simulink model "PresentationNetworkOrgignalparametrs3Copter"  (R2020a)
settings: Solver=FixedStepAuto  StartTime=0.0  StopTime=0.1  FixedStep=0.01  RelTol=1e-3
values from neighbouring files (symbols this model uses):
  Te = 0.012    [4двигателядообученный.mat]    (also in deepLearning.m; tdeepLearning.m)
  Tm = 0.025    [4двигателядообученный.mat]    (also in deepLearning.m; tdeepLearning.m)
  x1 = 1    [4двигателядообученный.mat]
  x2 = 1    [4двигателядообученный.mat]
  x3 = 1    [4двигателядообученный.mat]
undefined symbols (not defined in the file or in its folder): a1, a2, a3, a4, a5, b, d
libraries: simulink x3, dspsrcs4 x2, rllib x1
settings Model: Creator=xreno  LastModifiedBy=xreno

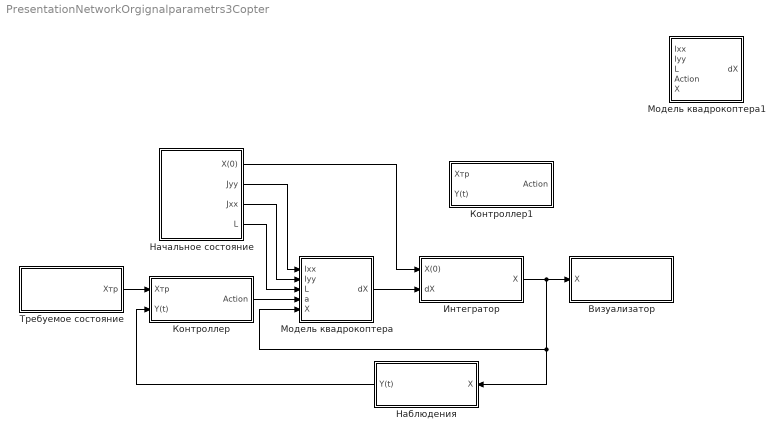
== system PresentationNetworkOrgignalparametrs3Copter ==
  Визуализатор : Subsystem
  Интегратор : Subsystem
  Контроллер : Subsystem
  Контроллер1 : Subsystem
  Модель квадрокоптера : Subsystem
  Модель квадрокоптера1 : Subsystem
  Наблюдения : Subsystem
  Начальное состояние : Subsystem
  Требуемое состояние : Subsystem
  wires:
  Начальное состояние/2(Jyy) -> Модель квадрокоптера/1(Ixx)
  Начальное состояние/1(X(0)) -> Интегратор/1(X(0))
  Модель квадрокоптера/1(dX) -> Интегратор/2(dX)
  Требуемое состояние/1(Xтр) -> Контроллер/1(Xтр)
  Интегратор/1(X) -> Наблюдения/1(X), Модель квадрокоптера/5(X), Визуализатор/1(X)
  Начальное состояние/3(Jxx) -> Модель квадрокоптера/2(Iyy)
  Наблюдения/1(Y(t)) -> Контроллер/2(Y(t))
  Начальное состояние/4(L) -> Модель квадрокоптера/3(L)
  Контроллер/1(Action) -> Модель квадрокоптера/4(a)

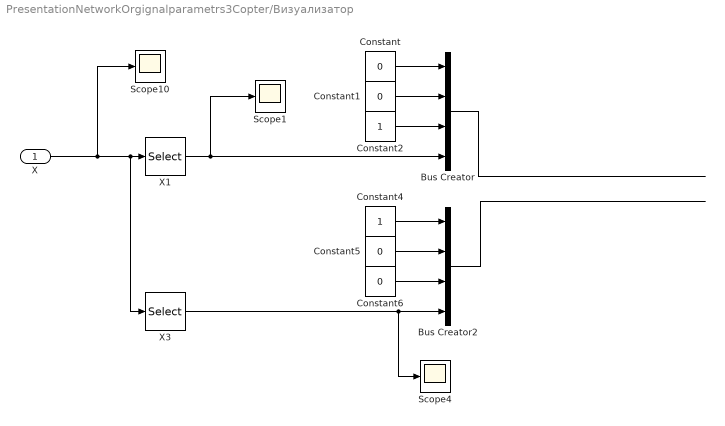
== system PresentationNetworkOrgignalparametrs3Copter/Визуализатор ==
  X : Inport
  Bus Creator : BusCreator  Inputs=4
  Bus Creator2 : BusCreator  Inputs=4
  Constant{,1,5..6} (4 alike) : Constant  Value=0
  Constant2 : Constant
  Constant4 : Constant
  Scope1 : Scope
  Scope10 : Scope
  Scope4 : Scope
  X1 : Selector  InputPortWidth=6  IndexOptions=Index vector (dialog)  Indices=[1]  OutputSizes=1
  X3 : Selector  InputPortWidth=6  IndexOptions=Index vector (dialog)  Indices=[3]  OutputSizes=1
  wires:
  Constant5/1 -> Bus Creator2/2
  Constant4/1 -> Bus Creator2/1
  Constant1/1 -> Bus Creator/2
  Bus Creator2/1 -> ?
  Constant6/1 -> Bus Creator2/3
  Constant2/1 -> Bus Creator/3
  Constant/1 -> Bus Creator/1
  Bus Creator/1 -> ?
  X/1 -> Scope10/1, X3/1, X1/1
  X1/1 -> Bus Creator/4, Scope1/1
  X3/1 -> Scope4/1, Bus Creator2/4

== system PresentationNetworkOrgignalparametrs3Copter/Интегратор ==
  X(0) : Inport
  dX : Inport  Port=2
  Integrator2 : Integrator  InitialConditionSource=external
  X : Outport
  wires:
  X(0)/1 -> Integrator2/2
  dX/1 -> Integrator2/1
  Integrator2/1 -> X/1

== system PresentationNetworkOrgignalparametrs3Copter/Контроллер ==
  Xтр : Inport
  Y(t) : Inport  Port=2
  Product2 : Product
  Rate Transition1 : RateTransition
  Rate Transition2 : RateTransition
  Rate Transition5 : RateTransition
  s1 : Constant  Value=8
  Блок RL Agent : rllib/RL Agent  Agent=agent  ProvideReward=on  ProvideIsDone=on  ProvideCumRwd=off  TreatAsDirectFeedthrough=on  CollectLoggedSignals=on  CollectModelStates=on
  Калькулятор награды : Subsystem
  Регулируемые параметры : Subsystem
  Action : Outport
  wires:
  Калькулятор награды/1(Reward) -> Rate Transition1/1
  Калькулятор награды/2(IsDone) -> Rate Transition2/1
  Product2/1 -> Action/1
  Регулируемые параметры/1(Z) -> Rate Transition5/1, Калькулятор награды/1(X)
  Блок RL Agent/1 -> Product2/2
  s1/1 -> Product2/1
  Rate Transition5/1 -> Блок RL Agent/1
  Rate Transition1/1 -> Блок RL Agent/2
  Rate Transition2/1 -> Блок RL Agent/3
  Y(t)/1 -> Регулируемые параметры/1(Y)
  Xтр/1 -> Регулируемые параметры/2(XT)

== system PresentationNetworkOrgignalparametrs3Copter/Контроллер1 ==
  Xтр : Inport
  Y(t) : Inport  Port=2
  Mux : Mux  Inputs=3
  PID-регулятор по крену : simulink/Continuous/PID Controller  Controller=PID  Form=Parallel  TimeDomain=Continuous-time  UseExternalTs=off  SampleTime=-1  IntegratorMethod=Forward Euler  FilterMethod=Forward Euler  ControllerParametersSource=internal  P=1  I=1  D=0  UseFilter=on  N=100  TunerSelectOption=Transfer Function Based (PID Tuner App)  InitialConditionSource=internal  InitialConditionForIntegrator=0  InitialConditionForFilter=0  DifferentiatorICPrevScaledInput=0  ExternalReset=none  TrackingMode=off  Kt=1  LimitOutput=off  UpperSaturationLimit=inf  LowerSaturationLimit=-inf  LinearizeAsGain=on  AntiWindupMode=none  Kb=1  POutMin=[]  POutMax=[]  IOutMin=[]  IOutMax=[]  DOutMin=[]  DOutMax=[]  NOutMin=[]  NOutMax=[]  SumOutMin=[]  SumOutMax=[]  SaturationOutMin=[]  SaturationOutMax=[]  PParamMin=[]  PParamMax=[]  IParamMin=[]  IParamMax=[]  DParamMin=[]  DParamMax=[]  NParamMin=[]  NParamMax=[]  KbParamMin=[]  KbParamMax=[]  KtParamMin=[]  KtParamMax=[]  KbOutMin=[]  KbOutMax=[]  KtOutMin=[]  KtOutMax=[]  IntegratorOutMin=[]  IntegratorOutMax=[]  FilterOutMin=[]  FilterOutMax=[]  SumI1OutMin=[]  SumI1OutMax=[]  SumI2OutMin=[]  SumI2OutMax=[]  SumI3OutMin=[]  SumI3OutMax=[]  SumI4OutMin=[]  SumI4OutMax=[]  SumDOutMin=[]  SumDOutMax=[]  DifferentiatorOutMin=[]  DifferentiatorOutMax=[]  FilterDiffOutCoefMin=[]  FilterDiffOutCoefMax=[]  ReciprocalOutMin=[]  ReciprocalOutMax=[]  SumDenOutMin=[]  SumDenOutMax=[]  SumNumOutMin=[]  SumNumOutMax=[]  DivideOutMin=[]  DivideOutMax=[]  UdiffTsProdOutMin=[]  UdiffTsProdOutMax=[]  NTsProdOutMin=[]  NTsProdOutMax=[]  UintegralTsProdOutMin=[]  UintegralTsProdOutMax=[]  UngainTsProdOutMin=[]  UngainTsProdOutMax=[]  IntegratorContinuousStateAttributes=''  IntegratorStateMustResolveToSignalObject=off  IntegratorRTWStateStorageClass=Auto  FilterContinuousStateAttributes=''  FilterStateMustResolveToSignalObject=off  FilterRTWStateStorageClass=Auto  ParallelPVariant=InternalParameters  IdealPVariant=Disabled  IVariant=InternalParameters  DVariant=InternalParameters  IntegratorVariant=Continuous  SatVariant=Disabled  AWVariant=Passthrough  PCopyVariant=Disabled  TRVariant=Disabled  FdbkBlocksVariant=Forward  IdealPFdbkVariant=Disabled  SatFdbkVariant=Disabled  DerivativeFilterVariant=ContFilter  NVariant=InternalParameters  NCopyVariant=Disabled  FilterICVariant=InternalICsFilter  IntegratorICVariant=InternalICs  ExternalResetVariant=Disabled  TRSumVariant=Passthrough  SumFdbkVariant=Disabled  SumVariant=Sum_PID  TsampFilterVariant=InternalTs  TsampNgainVariant=Passthrough  TsampIntegralVariant=Passthrough
  PID-регулятор по рысканью : simulink/Continuous/PID Controller  Controller=PID  Form=Parallel  TimeDomain=Continuous-time  UseExternalTs=off  SampleTime=-1  IntegratorMethod=Forward Euler  FilterMethod=Forward Euler  ControllerParametersSource=internal  P=1  I=1  D=0  UseFilter=on  N=100  TunerSelectOption=Transfer Function Based (PID Tuner App)  InitialConditionSource=internal  InitialConditionForIntegrator=0  InitialConditionForFilter=0  DifferentiatorICPrevScaledInput=0  ExternalReset=none  TrackingMode=off  Kt=1  LimitOutput=off  UpperSaturationLimit=inf  LowerSaturationLimit=-inf  LinearizeAsGain=on  AntiWindupMode=none  Kb=1  POutMin=[]  POutMax=[]  IOutMin=[]  IOutMax=[]  DOutMin=[]  DOutMax=[]  NOutMin=[]  NOutMax=[]  SumOutMin=[]  SumOutMax=[]  SaturationOutMin=[]  SaturationOutMax=[]  PParamMin=[]  PParamMax=[]  IParamMin=[]  IParamMax=[]  DParamMin=[]  DParamMax=[]  NParamMin=[]  NParamMax=[]  KbParamMin=[]  KbParamMax=[]  KtParamMin=[]  KtParamMax=[]  KbOutMin=[]  KbOutMax=[]  KtOutMin=[]  KtOutMax=[]  IntegratorOutMin=[]  IntegratorOutMax=[]  FilterOutMin=[]  FilterOutMax=[]  SumI1OutMin=[]  SumI1OutMax=[]  SumI2OutMin=[]  SumI2OutMax=[]  SumI3OutMin=[]  SumI3OutMax=[]  SumI4OutMin=[]  SumI4OutMax=[]  SumDOutMin=[]  SumDOutMax=[]  DifferentiatorOutMin=[]  DifferentiatorOutMax=[]  FilterDiffOutCoefMin=[]  FilterDiffOutCoefMax=[]  ReciprocalOutMin=[]  ReciprocalOutMax=[]  SumDenOutMin=[]  SumDenOutMax=[]  SumNumOutMin=[]  SumNumOutMax=[]  DivideOutMin=[]  DivideOutMax=[]  UdiffTsProdOutMin=[]  UdiffTsProdOutMax=[]  NTsProdOutMin=[]  NTsProdOutMax=[]  UintegralTsProdOutMin=[]  UintegralTsProdOutMax=[]  UngainTsProdOutMin=[]  UngainTsProdOutMax=[]  IntegratorContinuousStateAttributes=''  IntegratorStateMustResolveToSignalObject=off  IntegratorRTWStateStorageClass=Auto  FilterContinuousStateAttributes=''  FilterStateMustResolveToSignalObject=off  FilterRTWStateStorageClass=Auto  ParallelPVariant=InternalParameters  IdealPVariant=Disabled  IVariant=InternalParameters  DVariant=InternalParameters  IntegratorVariant=Continuous  SatVariant=Disabled  AWVariant=Passthrough  PCopyVariant=Disabled  TRVariant=Disabled  FdbkBlocksVariant=Forward  IdealPFdbkVariant=Disabled  SatFdbkVariant=Disabled  DerivativeFilterVariant=ContFilter  NVariant=InternalParameters  NCopyVariant=Disabled  FilterICVariant=InternalICsFilter  IntegratorICVariant=InternalICs  ExternalResetVariant=Disabled  TRSumVariant=Passthrough  SumFdbkVariant=Disabled  SumVariant=Sum_PID  TsampFilterVariant=InternalTs  TsampNgainVariant=Passthrough  TsampIntegralVariant=Passthrough
  PID-регулятор по тангажу : simulink/Continuous/PID Controller  Controller=PID  Form=Parallel  TimeDomain=Continuous-time  UseExternalTs=off  SampleTime=-1  IntegratorMethod=Forward Euler  FilterMethod=Forward Euler  ControllerParametersSource=internal  P=1  I=1  D=0  UseFilter=on  N=100  TunerSelectOption=Transfer Function Based (PID Tuner App)  InitialConditionSource=internal  InitialConditionForIntegrator=0  InitialConditionForFilter=0  DifferentiatorICPrevScaledInput=0  ExternalReset=none  TrackingMode=off  Kt=1  LimitOutput=off  UpperSaturationLimit=inf  LowerSaturationLimit=-inf  LinearizeAsGain=on  AntiWindupMode=none  Kb=1  POutMin=[]  POutMax=[]  IOutMin=[]  IOutMax=[]  DOutMin=[]  DOutMax=[]  NOutMin=[]  NOutMax=[]  SumOutMin=[]  SumOutMax=[]  SaturationOutMin=[]  SaturationOutMax=[]  PParamMin=[]  PParamMax=[]  IParamMin=[]  IParamMax=[]  DParamMin=[]  DParamMax=[]  NParamMin=[]  NParamMax=[]  KbParamMin=[]  KbParamMax=[]  KtParamMin=[]  KtParamMax=[]  KbOutMin=[]  KbOutMax=[]  KtOutMin=[]  KtOutMax=[]  IntegratorOutMin=[]  IntegratorOutMax=[]  FilterOutMin=[]  FilterOutMax=[]  SumI1OutMin=[]  SumI1OutMax=[]  SumI2OutMin=[]  SumI2OutMax=[]  SumI3OutMin=[]  SumI3OutMax=[]  SumI4OutMin=[]  SumI4OutMax=[]  SumDOutMin=[]  SumDOutMax=[]  DifferentiatorOutMin=[]  DifferentiatorOutMax=[]  FilterDiffOutCoefMin=[]  FilterDiffOutCoefMax=[]  ReciprocalOutMin=[]  ReciprocalOutMax=[]  SumDenOutMin=[]  SumDenOutMax=[]  SumNumOutMin=[]  SumNumOutMax=[]  DivideOutMin=[]  DivideOutMax=[]  UdiffTsProdOutMin=[]  UdiffTsProdOutMax=[]  NTsProdOutMin=[]  NTsProdOutMax=[]  UintegralTsProdOutMin=[]  UintegralTsProdOutMax=[]  UngainTsProdOutMin=[]  UngainTsProdOutMax=[]  IntegratorContinuousStateAttributes=''  IntegratorStateMustResolveToSignalObject=off  IntegratorRTWStateStorageClass=Auto  FilterContinuousStateAttributes=''  FilterStateMustResolveToSignalObject=off  FilterRTWStateStorageClass=Auto  ParallelPVariant=InternalParameters  IdealPVariant=Disabled  IVariant=InternalParameters  DVariant=InternalParameters  IntegratorVariant=Continuous  SatVariant=Disabled  AWVariant=Passthrough  PCopyVariant=Disabled  TRVariant=Disabled  FdbkBlocksVariant=Forward  IdealPFdbkVariant=Disabled  SatFdbkVariant=Disabled  DerivativeFilterVariant=ContFilter  NVariant=InternalParameters  NCopyVariant=Disabled  FilterICVariant=InternalICsFilter  IntegratorICVariant=InternalICs  ExternalResetVariant=Disabled  TRSumVariant=Passthrough  SumFdbkVariant=Disabled  SumVariant=Sum_PID  TsampFilterVariant=InternalTs  TsampNgainVariant=Passthrough  TsampIntegralVariant=Passthrough
  Scope : Scope
  Scope1 : Scope
  Selector1 : Selector  InputPortWidth=6  IndexOptions=Index vector (dialog)  Indices=[1]  OutputSizes=1
  Selector2 : Selector  InputPortWidth=6  IndexOptions=Index vector (dialog)  Indices=[3]  OutputSizes=1
  Selector3 : Selector  InputPortWidth=6  IndexOptions=Index vector (dialog)  Indices=[5]  OutputSizes=1
  Калькулятор награды : Subsystem
  Регулируемые параметры : Subsystem
  Action : Outport
  wires:
  Калькулятор награды/1(Reward) -> Scope/1
  Калькулятор награды/2(IsDone) -> Scope1/1
  Mux/1 -> Action/1
  Регулируемые параметры/1(Z) -> Калькулятор награды/1(X), Selector3/1, Selector1/1, Selector2/1
  Y(t)/1 -> Регулируемые параметры/1(Y)
  Xтр/1 -> Регулируемые параметры/2(XT)
  Selector1/1 -> PID-регулятор по крену/1
  Selector2/1 -> PID-регулятор по тангажу/1
  Selector3/1 -> PID-регулятор по рысканью/1
  PID-регулятор по тангажу/1 -> Mux/2
  PID-регулятор по крену/1 -> Mux/1
  PID-регулятор по рысканью/1 -> Mux/3

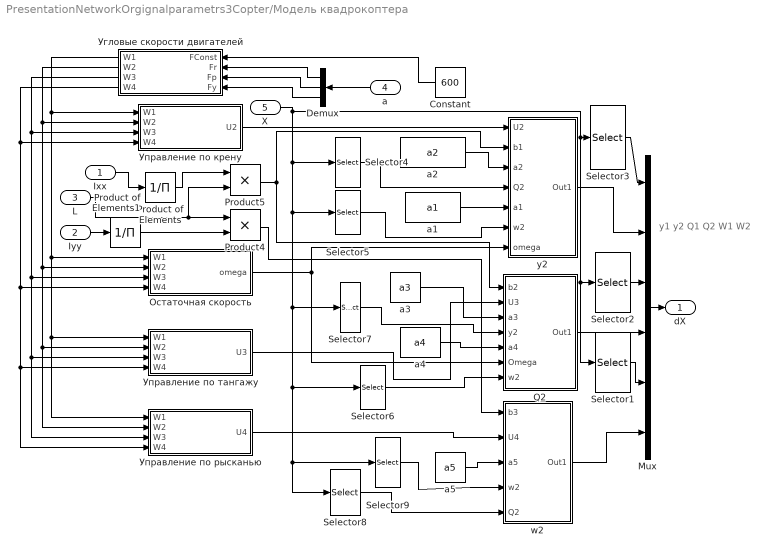
== system PresentationNetworkOrgignalparametrs3Copter/Модель квадрокоптера ==
  note: y1
      | y2
      | Q1
      | Q2
      | W1
      | W2
  Ixx : Inport
  Iyy : Inport  Port=2
  L : Inport  Port=3
  a : Inport  Port=4
  X : Inport  Port=5
  Constant : Constant  Value=600
  Demux : Demux  Outputs=3
  Mux : Mux  Inputs=6
  Product of Elements : Product  Inputs=/
  Product of Elements1 : Product  Inputs=/
  Product4 : Product
  Product5 : Product
  Q2 : Subsystem
  Selector{1,5..6,9} (4 alike) : Selector  InputPortWidth=6  IndexOptions=Index vector (dialog)  Indices=[6]  OutputSizes=1
  Selector2 : Selector  InputPortWidth=6  IndexOptions=Index vector (dialog)  Indices=[4]  OutputSizes=1
  Selector3 : Selector  InputPortWidth=6  IndexOptions=Index vector (dialog)  Indices=[2]  OutputSizes=1
  Selector4 : Selector  InputPortWidth=6  IndexOptions=Index vector (dialog)  Indices=[4]  OutputSizes=1
  Selector7 : Selector  InputPortWidth=6  IndexOptions=Index vector (dialog)  Indices=[2]  OutputSizes=1
  Selector8 : Selector  InputPortWidth=6  IndexOptions=Index vector (dialog)  Indices=[4]  OutputSizes=1
  a1 : Constant  Value=a1
  a2 : Constant  Value=a2
  a3 : Constant  Value=a3
  a4 : Constant  Value=a4
  a5 : Constant  Value=a5
  w2 : Subsystem
  y2 : Subsystem
  Остаточная скорость : Subsystem
  Угловые скорости двигателей : Subsystem
  Управление по крену : Subsystem
  Управление по рысканью : Subsystem
  Управление по тангажу : Subsystem
  dX : Outport
  wires:
  X/1 -> Selector3/1, Selector1/1, Selector2/1, Selector6/1, Selector9/1, Selector8/1, Selector7/1, Selector5/1, Selector4/1
  a/1 -> Demux/1
  Mux/1 -> dX/1
  Constant/1 -> Угловые скорости двигателей/1(FConst)
  Угловые скорости двигателей/2(W2) -> Управление по рысканью/2(W2), Управление по тангажу/2(W2), Остаточная скорость/2(W2), Управление по крену/2(W2)
  Угловые скорости двигателей/4(W4) -> Управление по рысканью/4(W4), Управление по тангажу/4(W4), Остаточная скорость/4(W4), Управление по крену/4(W4)
  Угловые скорости двигателей/3(W3) -> Управление по рысканью/3(W3), Управление по тангажу/3(W3), Остаточная скорость/3(W3), Управление по крену/3(W3)
  Управление по крену/1(U2) -> y2/1(U2)
  Product5/1 -> y2/2(b1), Q2/1(b2)
  Управление по тангажу/1(U3) -> Q2/2(U3)
  Product of Elements/1 -> Product5/1
  Product of Elements1/1 -> Product4/2
  Product4/1 -> w2/1(b3)
  L/1 -> Product5/2, Product4/1
  Iyy/1 -> Product of Elements1/1
  Ixx/1 -> Product of Elements/1
  Угловые скорости двигателей/1(W1) -> Управление по рысканью/1(W1), Управление по тангажу/1(W1), Остаточная скорость/1(W1), Управление по крену/1(W1)
  Demux/1 -> Угловые скорости двигателей/2(Fr)
  Demux/2 -> Угловые скорости двигателей/3(Fp)
  y2/1(Out1) -> Mux/2
  Q2/1(Out1) -> Mux/4
  w2/1(Out1) -> Mux/6
  Selector3/1 -> Mux/1
  Selector2/1 -> Mux/3
  Selector1/1 -> Mux/5
  Остаточная скорость/1(omega) -> y2/7(omega), Q2/6(Omega)
  a3/1 -> Q2/3(a3)
  a1/1 -> y2/5(a1)
  a2/1 -> y2/3(a2)
  a4/1 -> Q2/5(a4)
  a5/1 -> w2/3(a5)
  Управление по рысканью/1(U4) -> w2/2(U4)
  Selector4/1 -> y2/4(Q2)
  Selector5/1 -> y2/6(w2)
  Selector6/1 -> Q2/7(w2)
  Selector7/1 -> Q2/4(y2)
  Selector8/1 -> w2/5(Q2)
  Selector9/1 -> w2/4(w2)
  Demux/3 -> Угловые скорости двигателей/4(Fy)

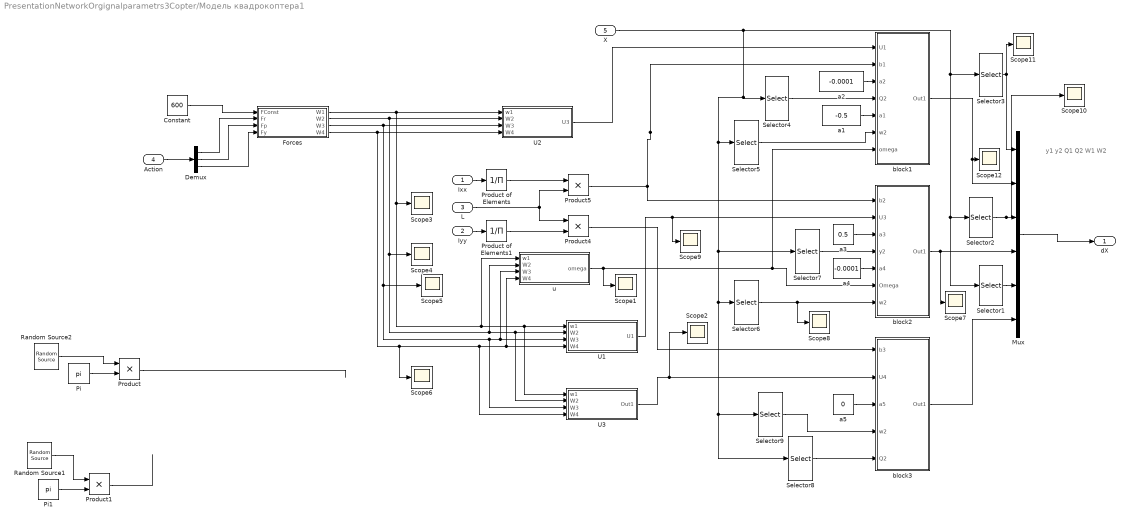
== system PresentationNetworkOrgignalparametrs3Copter/Модель квадрокоптера1 ==
  note: y1
      | y2
      | Q1
      | Q2
      | W1
      | W2
  Ixx : Inport
  Iyy : Inport  Port=2
  L : Inport  Port=3
  Action : Inport  Port=4
  X : Inport  Port=5
  Constant : Constant  Value=600
  Demux : Demux  Outputs=3
  Forces : Subsystem
  Mux : Mux  Inputs=6
  Pi : Constant  Value=pi  OutDataTypeStr=Inherit: Inherit via back propagation
  Pi1 : Constant  Value=pi  OutDataTypeStr=Inherit: Inherit via back propagation
  Product{,1,4..5} (4 alike) : Product
  Product of Elements : Product  Inputs=/
  Product of Elements1 : Product  Inputs=/
  Random Source1 : dspsrcs4/Random Source  SrcType=Uniform  NormMethod=Ziggurat  CltLength=12  MinVal=-1  MaxVal=1  MeanVal=0  VarVal=1  RepMode=Not repeatable  rawSeed=1  IsInherit=off  SampMode=Discrete  SampTime=1  SampFrame=1  DataType=Double  OutComplex=Real  OutputFrames=off
  Random Source2 : dspsrcs4/Random Source  SrcType=Uniform  NormMethod=Ziggurat  CltLength=12  MinVal=-1  MaxVal=1  MeanVal=0  VarVal=1  RepMode=Not repeatable  rawSeed=1  IsInherit=off  SampMode=Discrete  SampTime=1  SampFrame=1  DataType=Double  OutComplex=Real  OutputFrames=off
  Scope{1..12} (12 alike) : Scope
  Selector{1,5..6,9} (4 alike) : Selector  InputPortWidth=6  IndexOptions=Index vector (dialog)  Indices=[6]  OutputSizes=1
  Selector2 : Selector  InputPortWidth=6  IndexOptions=Index vector (dialog)  Indices=[4]  OutputSizes=1
  Selector3 : Selector  InputPortWidth=6  IndexOptions=Index vector (dialog)  Indices=[2]  OutputSizes=1
  Selector4 : Selector  InputPortWidth=6  IndexOptions=Index vector (dialog)  Indices=[4]  OutputSizes=1
  Selector7 : Selector  InputPortWidth=6  IndexOptions=Index vector (dialog)  Indices=[2]  OutputSizes=1
  Selector8 : Selector  InputPortWidth=6  IndexOptions=Index vector (dialog)  Indices=[4]  OutputSizes=1
  U1 : Subsystem
  U2 : Subsystem
  U3 : Subsystem
  a1 : Constant  Value=-0.5
  a2 : Constant  Value=-0.0001
  a3 : Constant  Value=0.5
  a4 : Constant  Value=-0.0001
  a5 : Constant  Value=0
  block1 : Subsystem
  block2 : Subsystem
  block3 : Subsystem
  u : Subsystem
  dX : Outport
  wires:
  X/1 -> Selector7/1, Selector8/1, Selector9/1, Selector6/1, Selector5/1, Selector4/1, Selector1/1, Selector2/1, Selector3/1
  Action/1 -> Demux/1
  Mux/1 -> dX/1
  Constant/1 -> Forces/1(FConst)
  Forces/2(W2) -> U2/2(W2), Scope4/1, u/2(W2), U1/2(W2), U3/2(W2)
  Forces/4(W4) -> U2/4(W4), Scope6/1, U3/4(W4), u/4(W4), U1/4(W4)
  Forces/3(W3) -> U2/3(W3), U3/3(W3), u/3(W3), U1/3(W3), Scope5/1
  U2/1(U3) -> block1/1(U1)
  Product5/1 -> block1/2(b1), block2/1(b2)
  U1/1(U1) -> Scope9/1, block2/2(U3)
  Product of Elements/1 -> Product5/1
  Product of Elements1/1 -> Product4/2
  Product4/1 -> block3/1(b3)
  L/1 -> Product4/1, Product5/2
  Iyy/1 -> Product of Elements1/1
  Ixx/1 -> Product of Elements/1
  Forces/1(W1) -> U2/1(w1), u/1(w1), U1/1(w1), U3/1(w1), Scope3/1
  Demux/1 -> Forces/2(Fr)
  Demux/2 -> Forces/3(Fp)
  block1/1(Out1) -> Scope12/1, Mux/2
  block2/1(Out1) -> Scope7/1, Mux/4
  block3/1(Out1) -> Mux/6
  Selector3/1 -> Scope11/1, Mux/1
  Selector2/1 -> Scope10/1, Mux/3
  Selector1/1 -> Mux/5
  u/1(omega) -> Scope1/1, block2/6(Omega), block1/7(omega)
  a3/1 -> block2/3(a3)
  a1/1 -> block1/5(a1)
  a2/1 -> block1/3(a2)
  a4/1 -> block2/5(a4)
  a5/1 -> block3/3(a5)
  U3/1(Out1) -> Scope2/1, block3/2(U4)
  Selector4/1 -> block1/4(Q2)
  Selector5/1 -> block1/6(w2)
  Selector6/1 -> Scope8/1, block2/7(w2)
  Selector7/1 -> block2/4(y2)
  Selector8/1 -> block3/5(Q2)
  Selector9/1 -> block3/4(w2)
  Demux/3 -> Forces/4(Fy)
  Pi1/1 -> Product1/2
  Product1/1 -> ?
  Pi/1 -> Product/2
  Random Source2/1 -> Product/1
  Random Source1/1 -> Product1/1
  Product/1 -> ?

== system PresentationNetworkOrgignalparametrs3Copter/Наблюдения ==
  X : Inport
  Demux : Demux  Outputs=6
  FucncN2 : MATLAB Function  TreatAsAtomicUnit=on
  FuncN1 : MATLAB Function  TreatAsAtomicUnit=on
  FuncN3 : MATLAB Function  TreatAsAtomicUnit=on
  Mux : Mux  Inputs=6
  Rate Transition{1,3..4,7} (4 alike) : RateTransition
  Y(t) : Outport
  wires:
  Mux/1 -> Y(t)/1
  Demux/3 -> FucncN2/1(inputArg1)
  FucncN2/1(outputArg1) -> Rate Transition1/1
  Rate Transition3/1 -> Mux/1
  Demux/2 -> Mux/2
  Demux/4 -> Mux/4
  X/1 -> Rate Transition4/1
  Rate Transition7/1 -> Mux/5
  Demux/5 -> FuncN3/1(inputArg1)
  Demux/6 -> Mux/6
  FuncN1/1(outputArg1) -> Rate Transition3/1
  Demux/1 -> FuncN1/1(inputArg1)
  Rate Transition4/1 -> Demux/1
  ? -> ?
  FuncN3/1(outputArg1) -> Rate Transition7/1
  Rate Transition1/1 -> Mux/3

== system PresentationNetworkOrgignalparametrs3Copter/Начальное состояние ==
  Constant1 : Constant  Value=0
  Constant2 : Constant  Value=x2
  Constant3 : Constant  Value=0
  Constant4 : Constant  Value=x1
  Constant5 : Constant  Value=x3
  Constant6 : Constant  Value=0
  Ixx : Constant
  Iyy : Constant
  L1 : Constant  Value=0.5
  Mux1 : Mux  Inputs=6
  X(0) : Outport
  Jyy : Outport  Port=2
  Jxx : Outport  Port=3
  L : Outport  Port=4
  wires:
  Constant1/1 -> Mux1/2
  Mux1/1 -> X(0)/1
  Constant3/1 -> Mux1/4
  Ixx/1 -> Jxx/1
  Iyy/1 -> Jyy/1
  L1/1 -> L/1
  Constant2/1 -> Mux1/3
  Constant4/1 -> Mux1/1
  Constant5/1 -> Mux1/5
  Constant6/1 -> Mux1/6

== system PresentationNetworkOrgignalparametrs3Copter/Требуемое состояние ==
  Constant{,1..5} (6 alike) : Constant  Value=0
  Mux1 : Mux  Inputs=6
  Xтр : Outport
  wires:
  Constant/1 -> Mux1/1
  Constant3/1 -> Mux1/4
  Constant1/1 -> Mux1/2
  Mux1/1 -> Xтр/1
  Constant2/1 -> Mux1/3
  Constant5/1 -> Mux1/6
  Constant4/1 -> Mux1/5

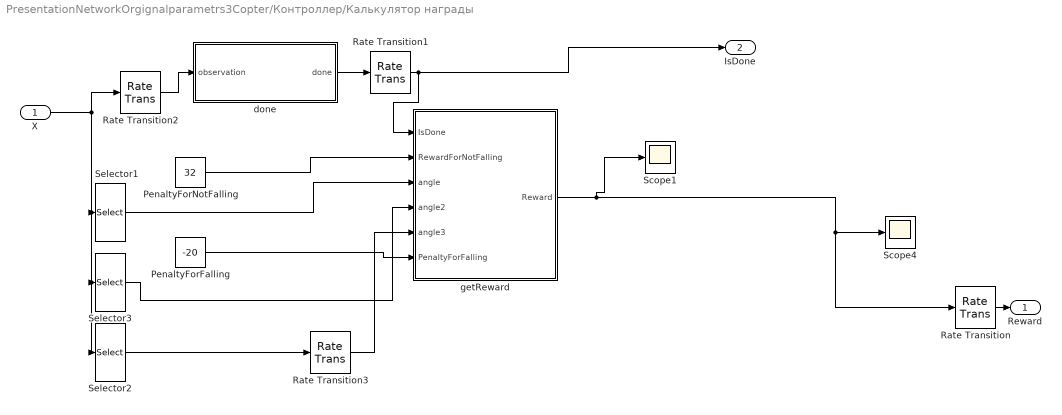
== system PresentationNetworkOrgignalparametrs3Copter/Контроллер/Калькулятор награды ==
  X : Inport
  PenaltyForFalling : Constant  Value=-20
  PenaltyForNotFalling : Constant  Value=32
  Rate Transition{,1..3} (4 alike) : RateTransition
  Scope1 : Scope
  Scope4 : Scope
  Selector1 : Selector  InputPortWidth=6  IndexOptions=Index vector (dialog)  Indices=[1]  OutputSizes=1
  Selector2 : Selector  InputPortWidth=6  IndexOptions=Index vector (dialog)  Indices=[5]  OutputSizes=1
  Selector3 : Selector  InputPortWidth=6  IndexOptions=Index vector (dialog)  Indices=[3]  OutputSizes=1
  done : MATLAB Function  TreatAsAtomicUnit=on
  getReward : MATLAB Function  TreatAsAtomicUnit=on
  Reward : Outport
  IsDone : Outport  Port=2
  wires:
  X/1 -> Rate Transition2/1, Selector2/1, Selector3/1, Selector1/1
  done/1(done) -> Rate Transition1/1
  getReward/1(Reward) -> Scope4/1, Rate Transition/1, Scope1/1
  Rate Transition/1 -> Reward/1
  Rate Transition2/1 -> done/1(observation)
  Rate Transition1/1 -> getReward/1(IsDone), IsDone/1
  PenaltyForNotFalling/1 -> getReward/2(RewardForNotFalling)
  Selector1/1 -> getReward/3(angle)
  PenaltyForFalling/1 -> getReward/6(PenaltyForFalling)
  Selector3/1 -> getReward/4(angle2)
  Selector2/1 -> Rate Transition3/1
  Rate Transition3/1 -> getReward/5(angle3)

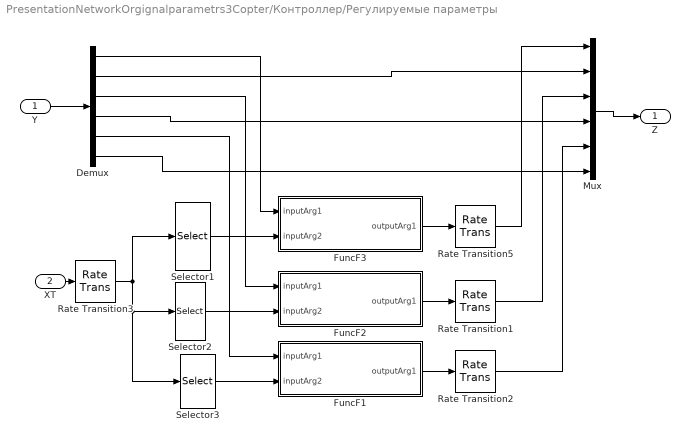
== system PresentationNetworkOrgignalparametrs3Copter/Контроллер/Регулируемые параметры ==
  Y : Inport
  XT : Inport  Port=2
  Demux : Demux  Outputs=6
  FuncF1 : MATLAB Function  TreatAsAtomicUnit=on
  FuncF2 : MATLAB Function  TreatAsAtomicUnit=on
  FuncF3 : MATLAB Function  TreatAsAtomicUnit=on
  Mux : Mux  Inputs=6
  Rate Transition{1..3,5} (4 alike) : RateTransition
  Selector1 : Selector  InputPortWidth=6  IndexOptions=Index vector (dialog)  Indices=[1]  OutputSizes=1
  Selector2 : Selector  InputPortWidth=6  IndexOptions=Index vector (dialog)  Indices=[3]  OutputSizes=1
  Selector3 : Selector  InputPortWidth=6  IndexOptions=Index vector (dialog)  Indices=[5]  OutputSizes=1
  Z : Outport
  wires:
  Mux/1 -> Z/1
  Y/1 -> Demux/1
  Demux/2 -> Mux/2
  Demux/4 -> Mux/4
  Demux/6 -> Mux/6
  Selector3/1 -> FuncF1/2(inputArg2)
  Rate Transition3/1 -> Selector1/1, Selector3/1, Selector2/1
  Demux/5 -> FuncF1/1(inputArg1)
  Rate Transition2/1 -> Mux/5
  Selector2/1 -> FuncF2/2(inputArg2)
  Rate Transition1/1 -> Mux/3
  Demux/3 -> FuncF2/1(inputArg1)
  Demux/1 -> FuncF3/1(inputArg1)
  Selector1/1 -> FuncF3/2(inputArg2)
  Rate Transition5/1 -> Mux/1
  FuncF3/1(outputArg1) -> Rate Transition5/1
  FuncF2/1(outputArg1) -> Rate Transition1/1
  FuncF1/1(outputArg1) -> Rate Transition2/1
  XT/1 -> Rate Transition3/1

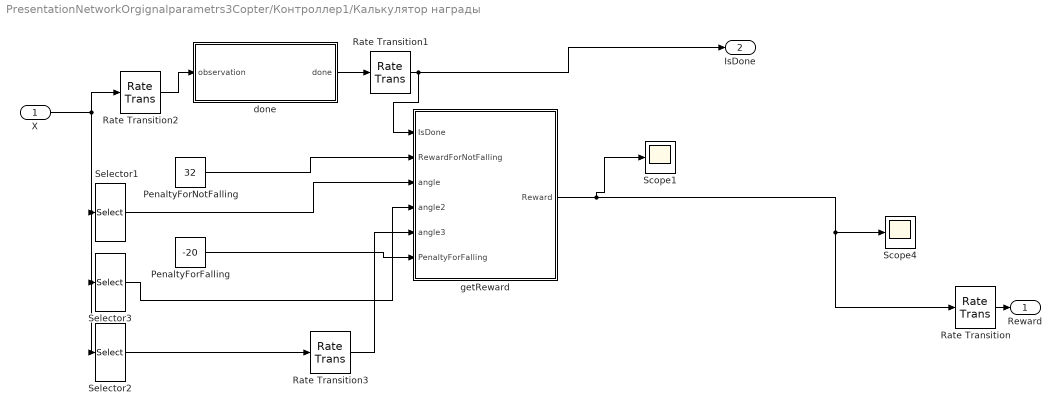
== system PresentationNetworkOrgignalparametrs3Copter/Контроллер1/Калькулятор награды ==
  X : Inport
  PenaltyForFalling : Constant  Value=-20
  PenaltyForNotFalling : Constant  Value=32
  Rate Transition{,1..3} (4 alike) : RateTransition
  Scope1 : Scope
  Scope4 : Scope
  Selector1 : Selector  InputPortWidth=6  IndexOptions=Index vector (dialog)  Indices=[1]  OutputSizes=1
  Selector2 : Selector  InputPortWidth=6  IndexOptions=Index vector (dialog)  Indices=[5]  OutputSizes=1
  Selector3 : Selector  InputPortWidth=6  IndexOptions=Index vector (dialog)  Indices=[3]  OutputSizes=1
  done : MATLAB Function  TreatAsAtomicUnit=on
  getReward : MATLAB Function  TreatAsAtomicUnit=on
  Reward : Outport
  IsDone : Outport  Port=2
  wires:
  X/1 -> Rate Transition2/1, Selector2/1, Selector3/1, Selector1/1
  done/1(done) -> Rate Transition1/1
  getReward/1(Reward) -> Scope4/1, Rate Transition/1, Scope1/1
  Rate Transition/1 -> Reward/1
  Rate Transition2/1 -> done/1(observation)
  Rate Transition1/1 -> getReward/1(IsDone), IsDone/1
  PenaltyForNotFalling/1 -> getReward/2(RewardForNotFalling)
  Selector1/1 -> getReward/3(angle)
  PenaltyForFalling/1 -> getReward/6(PenaltyForFalling)
  Selector3/1 -> getReward/4(angle2)
  Selector2/1 -> Rate Transition3/1
  Rate Transition3/1 -> getReward/5(angle3)

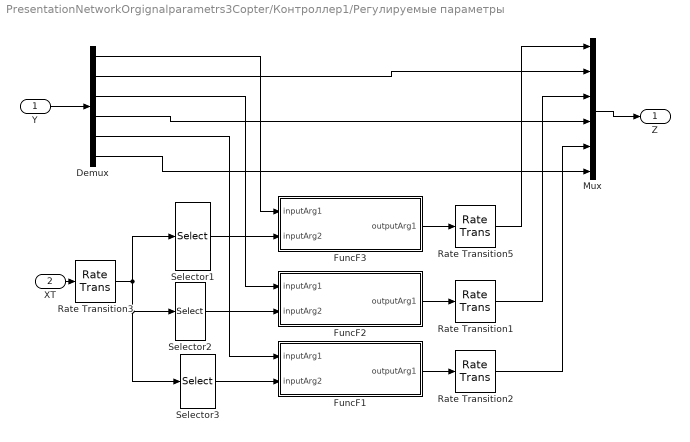
== system PresentationNetworkOrgignalparametrs3Copter/Контроллер1/Регулируемые параметры ==
  Y : Inport
  XT : Inport  Port=2
  Demux : Demux  Outputs=6
  FuncF1 : MATLAB Function  TreatAsAtomicUnit=on
  FuncF2 : MATLAB Function  TreatAsAtomicUnit=on
  FuncF3 : MATLAB Function  TreatAsAtomicUnit=on
  Mux : Mux  Inputs=6
  Rate Transition{1..3,5} (4 alike) : RateTransition
  Selector1 : Selector  InputPortWidth=6  IndexOptions=Index vector (dialog)  Indices=[1]  OutputSizes=1
  Selector2 : Selector  InputPortWidth=6  IndexOptions=Index vector (dialog)  Indices=[3]  OutputSizes=1
  Selector3 : Selector  InputPortWidth=6  IndexOptions=Index vector (dialog)  Indices=[5]  OutputSizes=1
  Z : Outport
  wires:
  Mux/1 -> Z/1
  Y/1 -> Demux/1
  Demux/2 -> Mux/2
  Demux/4 -> Mux/4
  Demux/6 -> Mux/6
  Selector3/1 -> FuncF1/2(inputArg2)
  Rate Transition3/1 -> Selector1/1, Selector3/1, Selector2/1
  Demux/5 -> FuncF1/1(inputArg1)
  Rate Transition2/1 -> Mux/5
  Selector2/1 -> FuncF2/2(inputArg2)
  Rate Transition1/1 -> Mux/3
  Demux/3 -> FuncF2/1(inputArg1)
  Demux/1 -> FuncF3/1(inputArg1)
  Selector1/1 -> FuncF3/2(inputArg2)
  Rate Transition5/1 -> Mux/1
  FuncF3/1(outputArg1) -> Rate Transition5/1
  FuncF2/1(outputArg1) -> Rate Transition1/1
  FuncF1/1(outputArg1) -> Rate Transition2/1
  XT/1 -> Rate Transition3/1

== system PresentationNetworkOrgignalparametrs3Copter/Модель квадрокоптера/Q2 ==
  b2 : Inport
  U3 : Inport  Port=2
  a3 : Inport  Port=3
  y2 : Inport  Port=4
  a4 : Inport  Port=5
  Omega : Inport  Port=6
  w2 : Inport  Port=7
  Plus1 : Sum  Inputs=+++
  Product1 : Product
  Product2 : Product  Inputs=3
  Product3 : Product  Inputs=3
  Out1 : Outport
  wires:
  b2/1 -> Product1/1
  U3/1 -> Product1/2
  Omega/1 -> Product2/1
  a4/1 -> Product2/3
  y2/1 -> Product3/1, Product2/2
  a3/1 -> Product3/2
  w2/1 -> Product3/3
  Product1/1 -> Plus1/1
  Product2/1 -> Plus1/2
  Product3/1 -> Plus1/3
  Plus1/1 -> Out1/1

== system PresentationNetworkOrgignalparametrs3Copter/Модель квадрокоптера/w2 ==
  b3 : Inport
  U4 : Inport  Port=2
  a5 : Inport  Port=3
  w2 : Inport  Port=4
  Q2 : Inport  Port=5
  Plus1 : Sum  Inputs=-+
  Product1 : Product
  Product3 : Product  Inputs=3
  Out1 : Outport
  wires:
  b3/1 -> Product1/1
  U4/1 -> Product1/2
  a5/1 -> Product3/2
  Product1/1 -> Plus1/1
  Product3/1 -> Plus1/2
  Plus1/1 -> Out1/1
  w2/1 -> Product3/3
  Q2/1 -> Product3/1

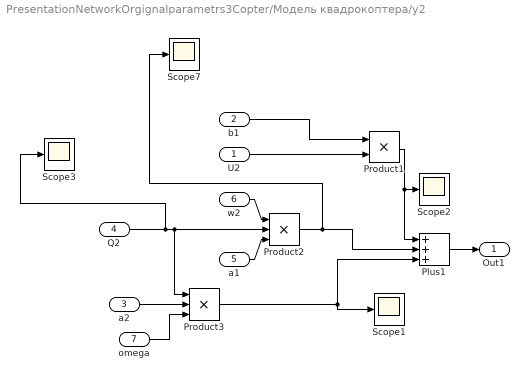
== system PresentationNetworkOrgignalparametrs3Copter/Модель квадрокоптера/y2 ==
  U2 : Inport
  b1 : Inport  Port=2
  a2 : Inport  Port=3
  Q2 : Inport  Port=4
  a1 : Inport  Port=5
  w2 : Inport  Port=6
  omega : Inport  Port=7
  Plus1 : Sum  Inputs=+++
  Product1 : Product
  Product2 : Product  Inputs=3
  Product3 : Product  Inputs=3
  Scope{1..3,7} (4 alike) : Scope
  Out1 : Outport
  wires:
  b1/1 -> Product1/1
  U2/1 -> Product1/2
  w2/1 -> Product2/1
  a1/1 -> Product2/3
  Q2/1 -> Scope3/1, Product3/1, Product2/2
  a2/1 -> Product3/2
  omega/1 -> Product3/3
  Product1/1 -> Scope2/1, Plus1/1
  Product2/1 -> Scope7/1, Plus1/2
  Product3/1 -> Plus1/3, Scope1/1
  Plus1/1 -> Out1/1

== system PresentationNetworkOrgignalparametrs3Copter/Модель квадрокоптера/Остаточная скорость ==
  W1 : Inport
  W2 : Inport  Port=2
  W3 : Inport  Port=3
  W4 : Inport  Port=4
  Add : Sum  Inputs=+--+
  omega : Outport
  wires:
  W1/1 -> Add/1
  W2/1 -> Add/2
  W3/1 -> Add/3
  W4/1 -> Add/4
  Add/1 -> omega/1

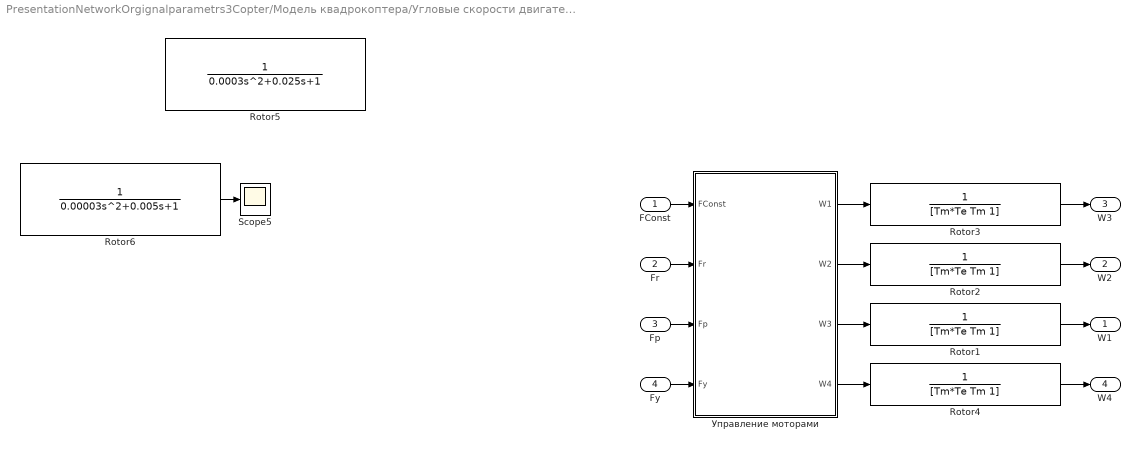
== system PresentationNetworkOrgignalparametrs3Copter/Модель квадрокоптера/Угловые скорости двигателей ==
  FConst : Inport
  Fr : Inport  Port=2
  Fp : Inport  Port=3
  Fy : Inport  Port=4
  Rotor{1..4} (4 alike) : TransferFcn  Denominator=[Tm*Te Tm 1]
  Rotor5 : TransferFcn  Denominator=[0.0003 0.025 1]
  Rotor6 : TransferFcn  Denominator=[0.00003 0.005 1]
  Scope5 : Scope
  Управление моторами : Subsystem
  W1 : Outport
  W2 : Outport  Port=2
  W3 : Outport  Port=3
  W4 : Outport  Port=4
  wires:
  FConst/1 -> Управление моторами/1(FConst)
  Управление моторами/4(W4) -> Rotor4/1
  Fy/1 -> Управление моторами/4(Fy)
  Rotor3/1 -> W3/1
  Rotor2/1 -> W2/1
  Rotor1/1 -> W1/1
  Rotor4/1 -> W4/1
  Rotor6/1 -> Scope5/1
  Fp/1 -> Управление моторами/3(Fp)
  Fr/1 -> Управление моторами/2(Fr)
  Управление моторами/1(W1) -> Rotor3/1
  Управление моторами/2(W2) -> Rotor2/1
  Управление моторами/3(W3) -> Rotor1/1

== system PresentationNetworkOrgignalparametrs3Copter/Модель квадрокоптера/Управление по крену ==
  W1 : Inport
  W2 : Inport  Port=2
  W3 : Inport  Port=3
  W4 : Inport  Port=4
  Add : Sum  Inputs=+-+-
  Product{,1..4} (5 alike) : Product
  b : Constant  Value=b
  U2 : Outport
  wires:
  W1/1 -> Product/2, Product/1
  W2/1 -> Product1/2, Product1/1
  W3/1 -> Product2/2, Product2/1
  W4/1 -> Product3/2, Product3/1
  Product/1 -> Add/1
  Product1/1 -> Add/2
  Product2/1 -> Add/3
  Product3/1 -> Add/4
  b/1 -> Product4/1
  Add/1 -> Product4/2
  Product4/1 -> U2/1

== system PresentationNetworkOrgignalparametrs3Copter/Модель квадрокоптера/Управление по рысканью ==
  W1 : Inport
  W2 : Inport  Port=2
  W3 : Inport  Port=3
  W4 : Inport  Port=4
  Add : Sum  Inputs=-++-
  Product{,1..4} (5 alike) : Product
  d : Constant  Value=d
  U4 : Outport
  wires:
  Add/1 -> Product4/2
  W4/1 -> Product3/2, Product3/1
  Product2/1 -> Add/3
  Product/1 -> Add/1
  W1/1 -> Product/2, Product/1
  Product1/1 -> Add/2
  W2/1 -> Product1/2, Product1/1
  W3/1 -> Product2/2, Product2/1
  Product3/1 -> Add/4
  d/1 -> Product4/1
  Product4/1 -> U4/1

== system PresentationNetworkOrgignalparametrs3Copter/Модель квадрокоптера/Управление по тангажу ==
  W1 : Inport
  W2 : Inport  Port=2
  W3 : Inport  Port=3
  W4 : Inport  Port=4
  Add : Sum  Inputs=++--
  Product{,1..4} (5 alike) : Product
  b : Constant  Value=b
  U3 : Outport
  wires:
  Add/1 -> Product4/2
  W4/1 -> Product3/2, Product3/1
  Product2/1 -> Add/3
  Product/1 -> Add/1
  W1/1 -> Product/2, Product/1
  Product1/1 -> Add/2
  W2/1 -> Product1/2, Product1/1
  W3/1 -> Product2/2, Product2/1
  Product3/1 -> Add/4
  b/1 -> Product4/1
  Product4/1 -> U3/1

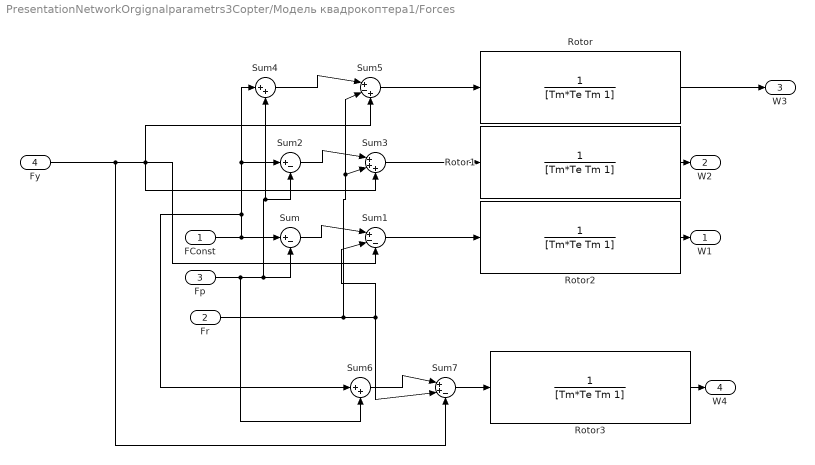
== system PresentationNetworkOrgignalparametrs3Copter/Модель квадрокоптера1/Forces ==
  FConst : Inport
  Fr : Inport  Port=2
  Fp : Inport  Port=3
  Fy : Inport  Port=4
  Rotor{,1..3} (4 alike) : TransferFcn  Denominator=[Tm*Te Tm 1]
  Sum : Sum  Inputs=|+-
  Sum1 : Sum  Inputs=|+--
  Sum2 : Sum  Inputs=|+-
  Sum3 : Sum  Inputs=|+++
  Sum4 : Sum  Inputs=|++
  Sum5 : Sum  Inputs=|+-+
  Sum6 : Sum  Inputs=|++
  Sum7 : Sum  Inputs=|++-
  W1 : Outport
  W2 : Outport  Port=2
  W3 : Outport  Port=3
  W4 : Outport  Port=4
  wires:
  Sum/1 -> Sum1/1
  Fp/1 -> Sum6/2, Sum4/2, Sum2/2, Sum/2
  Fr/1 -> Sum3/2, Sum5/2, Sum1/2, Sum7/2
  Sum2/1 -> Sum3/1
  Sum4/1 -> Sum5/1
  Sum6/1 -> Sum7/1
  FConst/1 -> Sum6/1, Sum4/1, Sum2/1, Sum/1
  Sum5/1 -> Rotor/1
  Sum7/1 -> Rotor3/1
  Sum1/1 -> Rotor2/1
  Sum3/1 -> Rotor1/1
  Fy/1 -> Sum1/3, Sum3/3, Sum5/3, Sum7/3
  Rotor/1 -> W3/1
  Rotor1/1 -> W2/1
  Rotor2/1 -> W1/1
  Rotor3/1 -> W4/1

== system PresentationNetworkOrgignalparametrs3Copter/Модель квадрокоптера1/U1 ==
  w1 : Inport
  W2 : Inport  Port=2
  W3 : Inport  Port=3
  W4 : Inport  Port=4
  Add : Sum  Inputs=++--
  Product{,1..4} (5 alike) : Product
  b : Constant  Value=0.001
  U1 : Outport
  wires:
  Add/1 -> Product4/2
  W4/1 -> Product3/2, Product3/1
  Product2/1 -> Add/3
  Product/1 -> Add/1
  w1/1 -> Product/2, Product/1
  Product1/1 -> Add/2
  W2/1 -> Product1/2, Product1/1
  W3/1 -> Product2/2, Product2/1
  Product3/1 -> Add/4
  b/1 -> Product4/1
  Product4/1 -> U1/1

== system PresentationNetworkOrgignalparametrs3Copter/Модель квадрокоптера1/U2 ==
  w1 : Inport
  W2 : Inport  Port=2
  W3 : Inport  Port=3
  W4 : Inport  Port=4
  Add : Sum  Inputs=+-+-
  Product{,1..4} (5 alike) : Product
  b : Constant  Value=0.001
  U3 : Outport
  wires:
  w1/1 -> Product/2, Product/1
  W2/1 -> Product1/2, Product1/1
  W3/1 -> Product2/2, Product2/1
  W4/1 -> Product3/2, Product3/1
  Product/1 -> Add/1
  Product1/1 -> Add/2
  Product2/1 -> Add/3
  Product3/1 -> Add/4
  b/1 -> Product4/1
  Add/1 -> Product4/2
  Product4/1 -> U3/1

== system PresentationNetworkOrgignalparametrs3Copter/Модель квадрокоптера1/U3 ==
  w1 : Inport
  W2 : Inport  Port=2
  W3 : Inport  Port=3
  W4 : Inport  Port=4
  Add : Sum  Inputs=-++-
  Product{,1..4} (5 alike) : Product
  b1 : Constant  Value=0.0008
  Out1 : Outport
  wires:
  Add/1 -> Product4/2
  W4/1 -> Product3/2, Product3/1
  Product2/1 -> Add/3
  Product/1 -> Add/1
  w1/1 -> Product/2, Product/1
  Product1/1 -> Add/2
  W2/1 -> Product1/2, Product1/1
  W3/1 -> Product2/2, Product2/1
  Product3/1 -> Add/4
  b1/1 -> Product4/1
  Product4/1 -> Out1/1

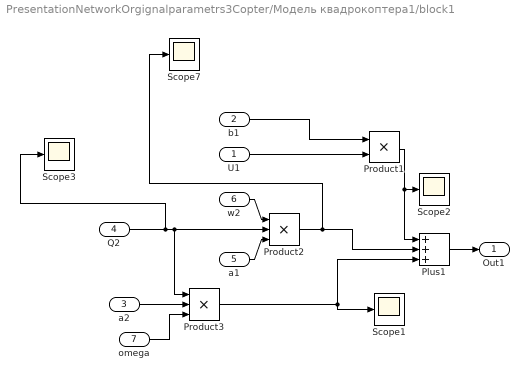
== system PresentationNetworkOrgignalparametrs3Copter/Модель квадрокоптера1/block1 ==
  U1 : Inport
  b1 : Inport  Port=2
  a2 : Inport  Port=3
  Q2 : Inport  Port=4
  a1 : Inport  Port=5
  w2 : Inport  Port=6
  omega : Inport  Port=7
  Plus1 : Sum  Inputs=+++
  Product1 : Product
  Product2 : Product  Inputs=3
  Product3 : Product  Inputs=3
  Scope{1..3,7} (4 alike) : Scope
  Out1 : Outport
  wires:
  b1/1 -> Product1/1
  U1/1 -> Product1/2
  w2/1 -> Product2/1
  a1/1 -> Product2/3
  Q2/1 -> Scope3/1, Product3/1, Product2/2
  a2/1 -> Product3/2
  omega/1 -> Product3/3
  Product1/1 -> Scope2/1, Plus1/1
  Product2/1 -> Scope7/1, Plus1/2
  Product3/1 -> Plus1/3, Scope1/1
  Plus1/1 -> Out1/1

== system PresentationNetworkOrgignalparametrs3Copter/Модель квадрокоптера1/block2 ==
  b2 : Inport
  U3 : Inport  Port=2
  a3 : Inport  Port=3
  y2 : Inport  Port=4
  a4 : Inport  Port=5
  Omega : Inport  Port=6
  w2 : Inport  Port=7
  Plus1 : Sum  Inputs=+++
  Product1 : Product
  Product2 : Product  Inputs=3
  Product3 : Product  Inputs=3
  Out1 : Outport
  wires:
  b2/1 -> Product1/1
  U3/1 -> Product1/2
  Omega/1 -> Product2/1
  a4/1 -> Product2/3
  y2/1 -> Product3/1, Product2/2
  a3/1 -> Product3/2
  w2/1 -> Product3/3
  Product1/1 -> Plus1/1
  Product2/1 -> Plus1/2
  Product3/1 -> Plus1/3
  Plus1/1 -> Out1/1

== system PresentationNetworkOrgignalparametrs3Copter/Модель квадрокоптера1/block3 ==
  b3 : Inport
  U4 : Inport  Port=2
  a5 : Inport  Port=3
  w2 : Inport  Port=4
  Q2 : Inport  Port=5
  Plus1 : Sum  Inputs=-+
  Product1 : Product
  Product3 : Product  Inputs=3
  Out1 : Outport
  wires:
  b3/1 -> Product1/1
  U4/1 -> Product1/2
  a5/1 -> Product3/2
  Product1/1 -> Plus1/1
  Product3/1 -> Plus1/2
  Plus1/1 -> Out1/1
  w2/1 -> Product3/3
  Q2/1 -> Product3/1

== system PresentationNetworkOrgignalparametrs3Copter/Модель квадрокоптера1/u ==
  w1 : Inport
  W2 : Inport  Port=2
  W3 : Inport  Port=3
  W4 : Inport  Port=4
  Add : Sum  Inputs=+--+
  omega : Outport
  wires:
  w1/1 -> Add/1
  W2/1 -> Add/2
  W3/1 -> Add/3
  W4/1 -> Add/4
  Add/1 -> omega/1

== system PresentationNetworkOrgignalparametrs3Copter/Модель квадрокоптера/Угловые скорости двигателей/Управление моторами ==
  FConst : Inport
  Fr : Inport  Port=2
  Fp : Inport  Port=3
  Fy : Inport  Port=4
  Add : Sum  Inputs=+++-
  Add1 : Sum  Inputs=+-++
  Add2 : Sum  Inputs=+---
  Add3 : Sum  Inputs=++-+
  W1 : Outport
  W2 : Outport  Port=2
  W3 : Outport  Port=3
  W4 : Outport  Port=4
  wires:
  Fp/1 -> Add3/1, Add1/2, Add/2, Add2/2
  Fy/1 -> Add3/3, Add2/3, Add1/3, Add/3
  Fr/1 -> Add/4, Add1/4, Add2/4, Add3/4
  FConst/1 -> Add2/1, Add3/2, Add1/1, Add/1
  Add/1 -> W3/1
  Add1/1 -> W2/1
  Add2/1 -> W1/1
  Add3/1 -> W4/1

== matlab function PresentationNetworkOrgignalparametrs3Copter/Контроллер/Калькулятор награды/getReward ==
  data: IsDone input; Reward output; RewardForNotFalling input; angle input; angle2 input; angle3 input; PenaltyForFalling input
       function Reward = getReward(IsDone, RewardForNotFalling, angle, angle2, angle3, PenaltyForFalling )
            if (IsDone ==0)
                

                Reward=RewardForNotFalling/(abs(angle)+abs(angle2)+abs(angle3)+0.001);

                
                   
                    
            else
                Reward = PenaltyForFalling;
            end 
            
        end

== matlab function PresentationNetworkOrgignalparametrs3Copter/Контроллер1/Регулируемые параметры/FuncF2 ==
  data: outputArg1 output; inputArg1 input; inputArg2 input
function outputArg1 = Angle12(inputArg1,inputArg2)
            %UNTITLED Summary of this function goes here
            % Detailed explanation goes here
            X = inputArg1-inputArg2;
            outputArg1=0;
            
            if (X<-pi)
                outputArg1=X+2*pi;
            end
            if (X>pi)
                outputArg1=X-2*pi;
            end
            if ((X<=pi)&&(X>=-pi))
                outputArg1=X;
            end
            
        end

== matlab function PresentationNetworkOrgignalparametrs3Copter/Контроллер1/Регулируемые параметры/FuncF3 ==
  data: outputArg1 output; inputArg1 input; inputArg2 input
function outputArg1 = Angle12(inputArg1,inputArg2)
            %UNTITLED Summary of this function goes here
            % Detailed explanation goes here
            X = inputArg1-inputArg2;
            outputArg1=0;
            
            if (X<-pi)
                outputArg1=X+2*pi;
            end
            if (X>pi)
                outputArg1=X-2*pi;
            end
            if ((X<=pi)&&(X>=-pi))
                outputArg1=X;
            end
            
        end

== matlab function PresentationNetworkOrgignalparametrs3Copter/Контроллер/Регулируемые параметры/FuncF1 ==
  data: outputArg1 output; inputArg1 input; inputArg2 input
function outputArg1 = Angle12(inputArg1,inputArg2)
            %UNTITLED Summary of this function goes here
            % Detailed explanation goes here
            X = inputArg1-inputArg2;
            outputArg1=0;
            
            if (X<-pi)
                outputArg1=X+2*pi;
            end
            if (X>pi)
                outputArg1=X-2*pi;
            end
            if ((X<=pi)&&(X>=-pi))
                outputArg1=X;
            end
            
        end

== matlab function PresentationNetworkOrgignalparametrs3Copter/Контроллер/Регулируемые параметры/FuncF2 ==
  data: outputArg1 output; inputArg1 input; inputArg2 input
function outputArg1 = Angle12(inputArg1,inputArg2)
            %UNTITLED Summary of this function goes here
            % Detailed explanation goes here
            X = inputArg1-inputArg2;
            outputArg1=0;
            
            if (X<-pi)
                outputArg1=X+2*pi;
            end
            if (X>pi)
                outputArg1=X-2*pi;
            end
            if ((X<=pi)&&(X>=-pi))
                outputArg1=X;
            end
            
        end

== matlab function PresentationNetworkOrgignalparametrs3Copter/Контроллер1/Калькулятор награды/done ==
  settings: updateMethod=DISCRETE
  data: observation input; done output
       function done = isDone(observation)
       done = ((abs(observation(2))>5)||(abs(observation(4))>5)||(abs(observation(6))>5));
       end

== matlab function PresentationNetworkOrgignalparametrs3Copter/Контроллер1/Калькулятор награды/getReward ==
  data: IsDone input; Reward output; RewardForNotFalling input; angle input; angle2 input; angle3 input; PenaltyForFalling input
       function Reward = getReward(IsDone, RewardForNotFalling, angle, angle2, angle3, PenaltyForFalling )
            if (IsDone ==0)
                

                Reward=RewardForNotFalling/(abs(angle)+abs(angle2)+abs(angle3)+0.001);

                
                   
                    
            else
                Reward = PenaltyForFalling;
            end 
            
        end

== matlab function PresentationNetworkOrgignalparametrs3Copter/Наблюдения/FuncN1 ==
  data: outputArg1 output; inputArg1 input
        function outputArg1 = angle(inputArg1)
            %ANGLE Summary of this function goes here
            % Detailed explanation goes here
            outputArg1=0;
            outputArg1=inputArg1;
            if(inputArg1<0)
                outputArg1 = pi*2+inputArg1;
            end
            if(inputArg1>2*pi)
                outputArg1 = -pi*2+inputArg1;
            end
            
        end

== matlab function PresentationNetworkOrgignalparametrs3Copter/Наблюдения/FucncN2 ==
  data: outputArg1 output; inputArg1 input
        function outputArg1 = angle(inputArg1)
            %ANGLE Summary of this function goes here
            % Detailed explanation goes here
            outputArg1 = 0;
            
            outputArg1=inputArg1;
            if(inputArg1<0)
                outputArg1 = pi*2+inputArg1;
            end
            if(inputArg1>2*pi)
                outputArg1 = -pi*2+inputArg1;
            end
            
        end

== matlab function PresentationNetworkOrgignalparametrs3Copter/Контроллер1/Регулируемые параметры/FuncF1 ==
  data: outputArg1 output; inputArg1 input; inputArg2 input
function outputArg1 = Angle12(inputArg1,inputArg2)
            %UNTITLED Summary of this function goes here
            % Detailed explanation goes here
            X = inputArg1-inputArg2;
            outputArg1=0;
            
            if (X<-pi)
                outputArg1=X+2*pi;
            end
            if (X>pi)
                outputArg1=X-2*pi;
            end
            if ((X<=pi)&&(X>=-pi))
                outputArg1=X;
            end
            
        end

== matlab function PresentationNetworkOrgignalparametrs3Copter/Наблюдения/FuncN3 ==
  data: outputArg1 output; inputArg1 input
        function outputArg1 = angle(inputArg1)
            %ANGLE Summary of this function goes here
            % Detailed explanation goes here
            outputArg1=0;
            outputArg1=inputArg1;
            if(inputArg1<0)
                outputArg1 = pi*2+inputArg1;
            end
            if(inputArg1>2*pi)
                outputArg1 = -pi*2+inputArg1;
            end
            
        end

== matlab function PresentationNetworkOrgignalparametrs3Copter/Контроллер/Калькулятор награды/done ==
  settings: updateMethod=DISCRETE
  data: observation input; done output
       function done = isDone(observation)
       done = ((abs(observation(2))>5)||(abs(observation(4))>5)||(abs(observation(6))>5));
       end

== matlab function PresentationNetworkOrgignalparametrs3Copter/Контроллер/Регулируемые параметры/FuncF3 ==
  data: outputArg1 output; inputArg1 input; inputArg2 input
function outputArg1 = Angle12(inputArg1,inputArg2)
            %UNTITLED Summary of this function goes here
            % Detailed explanation goes here
            X = inputArg1-inputArg2;
            outputArg1=0;
            
            if (X<-pi)
                outputArg1=X+2*pi;
            end
            if (X>pi)
                outputArg1=X-2*pi;
            end
            if ((X<=pi)&&(X>=-pi))
                outputArg1=X;
            end
            
        end
